simulink model "dsm_o2_scaling_system"  (R2021b)
settings: Solver=VariableStepAuto  StartTime=0.0  StopTime=t_sim - 1/51.2e6  RelTol=1e-3
undefined symbols (not defined in the file): a1, a2, b1, b2, c1, c2, f, f_sampling, vin
libraries: simulink_extras x2
settings Model: Creator=Raymond.Yang  LastModifiedBy=Raymond.Yang
settings SolverCC: AlgebraicLoopSolver=TrustRegion
settings DebuggingCC: SFMachineParentedDataDiag=warning

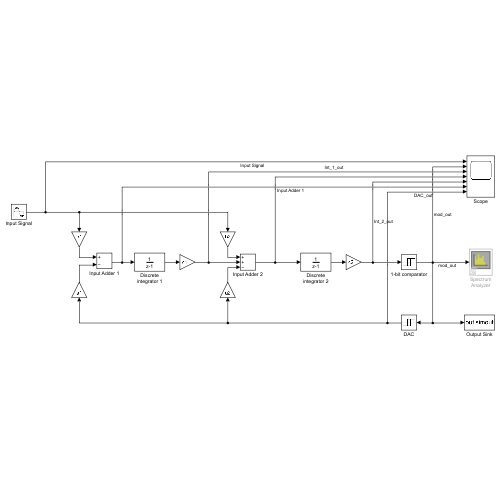
[thumbnail: Simulink's stored preview of the top-level diagram]
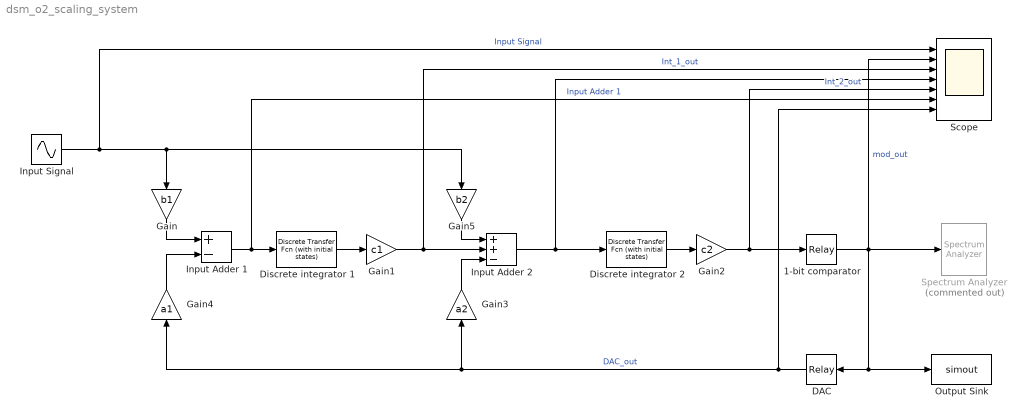
== system dsm_o2_scaling_system ==
  1-bit comparator : Relay  OnSwitchValue=0  OffSwitchValue=0  OffOutputValue=-1
  DAC : Relay  OnSwitchValue=1  OffSwitchValue=-1  OnOutputValue=vref_p  OffOutputValue=vref_n
  Discrete integrator 1 : simulink_extras/Additional Discrete/Discrete Transfer Fcn (with initial states)  N=[1]  D="[1  -1]"  X0=0  TS=-1
      settings: SourceProductBaseCode=SL
  Discrete integrator 2 : simulink_extras/Additional Discrete/Discrete Transfer Fcn (with initial states)  N=[1]  D="[1  -1]"  X0=0  TS=-1
      settings: SourceProductBaseCode=SL
  Gain : Gain  Gain=b1
  Gain1 : Gain  Gain=c1
  Gain2 : Gain  Gain=c2
  Gain3 : Gain  Gain=a2
  Gain4 : Gain  Gain=a1
  Gain5 : Gain  Gain=b2
  Input Adder 1 : Sum  Inputs=+-
  "Input Adder 2 " : Sum  Inputs=++-
  Input Signal : Sin  Amplitude=vin  Frequency=f*2*pi  SampleTime=1/(f_sampling)
  "Output Sink " : ToWorkspace  VariableName=simout  SaveFormat=Timeseries  SampleTime=-1
  Scope : Scope  NumInputPorts=7
  Spectrum Analyzer : SpectrumAnalyzer  Commented=on
  wires:
  DAC/1 -> Gain4/1, Gain3/1, Scope/7  "DAC_out"
  1-bit comparator/1 -> Scope/2, DAC/1, "Output Sink "/1, Spectrum Analyzer/1  "mod_out"
  Input Adder 1/1 -> Scope/6, Discrete integrator 1/1  "Input Adder 1"
  Discrete integrator 1/1 -> Gain1/1
  Input Signal/1 -> Gain/1, Gain5/1, Scope/1  "Input Signal"
  Gain/1 -> Input Adder 1/1
  Gain1/1 -> "Input Adder 2 "/2, Scope/3  "Int_1_out"
  Discrete integrator 2/1 -> Gain2/1
  Gain3/1 -> "Input Adder 2 "/3
  Gain4/1 -> Input Adder 1/2
  "Input Adder 2 "/1 -> Discrete integrator 2/1, Scope/4
  Gain2/1 -> 1-bit comparator/1, Scope/5  "Int_2_out"
  Gain5/1 -> "Input Adder 2 "/1
